simulink model "real_model_ctrl_2023a"  (R2024b)
settings: Solver=VariableStepAuto  StartTime=0.0  StopTime=1000  RelTol=1e-3
undefined symbols (not defined in the file or in its folder): National_Instruments, PCI
libraries: sldrtlib x3, slpidlib x1
settings Model: Creator=andit  LastModifiedBy=andit

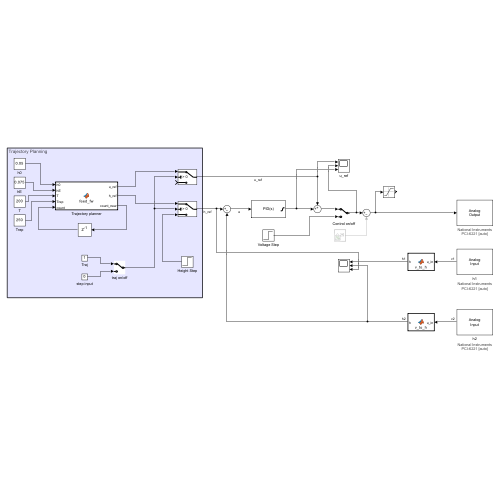
[thumbnail: Simulink's stored preview of the top-level diagram]
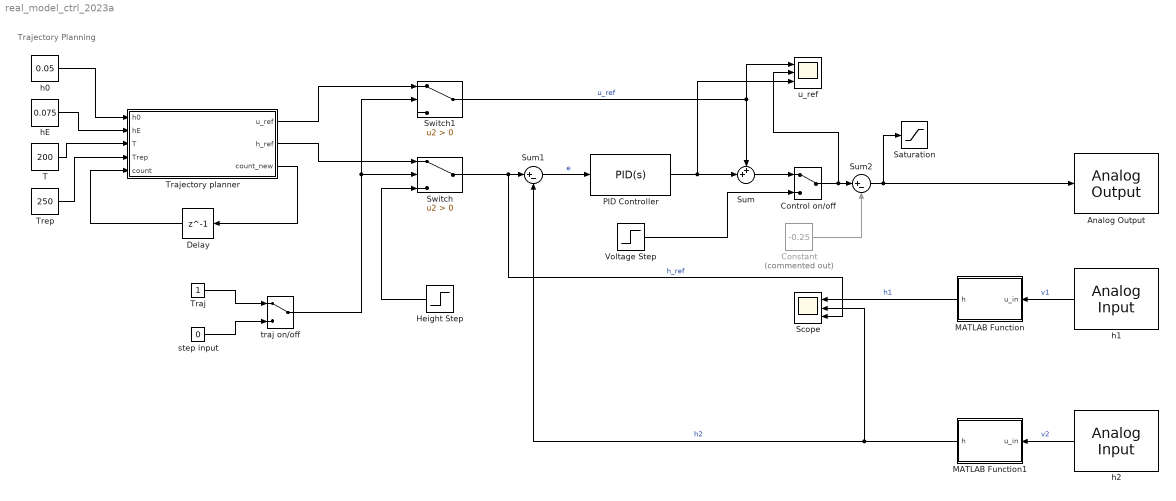
== system real_model_ctrl_2023a ==
  note: Trajectory Planning
  Analog Output : sldrtlib/Analog Output  SampleTime=0.1  MaxMissedTicks=10  ShowMissedTicks=off  YieldWhenWaiting=off  DrvName=National_Instruments/PCI-6221  DrvAddress=4294967295  DrvOptions=[0 1 0 0 0]  Channels=1  RangeMode=1  VoltRange=1  InitialValue=[]  FinalValue=[]
      settings: AttributesFormatString=National Instruments\nPCI-6221 [auto]
  Constant : Constant  Commented=on  Value=-0.25
  Control on/off : ManualSwitch
  Delay : Delay  DelayLength=1
  Height Step : Step  After=50  SampleTime=0
  MATLAB Function : MATLAB Function  TreatAsAtomicUnit=on
  MATLAB Function1 : MATLAB Function  TreatAsAtomicUnit=on
  PID Controller : slpidlib/PID Controller  Controller=PID  Form=Parallel  TimeDomain=Continuous-time  UseExternalTs=off  SampleTime=-1  IntegratorMethod=Forward Euler  FilterMethod=Forward Euler  ControllerParametersSource=internal  P=20  I=5  UseKiTs=off  D=-0.145290491513972  UseExternalDerivativeSource=off  N=13.0234851937353  UseFilter=on  TunerSelectOption=Transfer Function Based (PID Tuner App)  InitialConditionSource=internal  InitialConditionForIntegrator=0  InitialConditionForFilter=0  DifferentiatorICPrevScaledInput=0  ExternalReset=none  TrackingMode=off  Kt=1  LimitOutput=on  SatLimitsSource=internal  UpperSaturationLimit=5  LowerSaturationLimit=0  LinearizeAsGain=on  AntiWindupMode=clamping  Kb=1  LimitIntegrator=off  UpperIntegratorSaturationLimit=inf  LowerIntegratorSaturationLimit=-inf  POutMin=[]  POutMax=[]  IOutMin=[]  IOutMax=[]  DOutMin=[]  DOutMax=[]  NOutMin=[]  NOutMax=[]  SumOutMin=[]  SumOutMax=[]  SaturationOutMin=[]  SaturationOutMax=[]  PParamMin=[]  PParamMax=[]  IParamMin=[]  IParamMax=[]  DParamMin=[]  DParamMax=[]  NParamMin=[]  NParamMax=[]  KbParamMin=[]  KbParamMax=[]  KtParamMin=[]  KtParamMax=[]  KbOutMin=[]  KbOutMax=[]  KtOutMin=[]  KtOutMax=[]  IntegratorOutMin=[]  IntegratorOutMax=[]  FilterOutMin=[]  FilterOutMax=[]  SumI1OutMin=[]  SumI1OutMax=[]  SumI2OutMin=[]  SumI2OutMax=[]  SumI3OutMin=[]  SumI3OutMax=[]  SumI4OutMin=[]  SumI4OutMax=[]  SumDOutMin=[]  SumDOutMax=[]  DifferentiatorOutMin=[]  DifferentiatorOutMax=[]  FilterDiffOutCoefMin=[]  FilterDiffOutCoefMax=[]  ReciprocalOutMin=[]  ReciprocalOutMax=[]  SumDenOutMin=[]  SumDenOutMax=[]  SumNumOutMin=[]  SumNumOutMax=[]  DivideOutMin=[]  DivideOutMax=[]  UdiffTsProdOutMin=[]  UdiffTsProdOutMax=[]  NTsProdOutMin=[]  NTsProdOutMax=[]  UintegralTsProdOutMin=[]  UintegralTsProdOutMax=[]  UngainTsProdOutMin=[]  UngainTsProdOutMax=[]  ClampingZeroOutDataTypeStr=Inherit: Inherit via back propagation  ClampingZeroOutMin=[]  ClampingZeroOutMax=[]  FilterDenConstantOutDataTypeStr=Inherit: Inherit via back propagation  FilterDenConstantOutMin=[]  FilterDenConstantOutMax=[]  PCopyOutDataTypeStr=Inherit: Inherit via back propagation  PCopyOutMin=[]  PCopyOutMax=[]  NCopyOutDataTypeStr=Inherit: Inherit via back propagation  NCopyOutMin=[]  NCopyOutMax=[]  IntegratorContinuousStateAttributes=''  IntegratorStateMustResolveToSignalObject=off  IntegratorRTWStateStorageClass=Auto  FilterContinuousStateAttributes=''  FilterStateMustResolveToSignalObject=off  FilterRTWStateStorageClass=Auto  ParallelPVariant=InternalParameters  IdealPVariant=Disabled  IVariant=InternalParameters  DVariant=InternalParameters  IntegratorVariant=Continuous  SatVariant=Enabled  AWVariant=ContClampingParallel  PCopyVariant=Disabled  TRVariant=Disabled  FdbkBlocksVariant=Forward  IdealPFdbkVariant=Disabled  SatFdbkVariant=Disabled  DerivativeFilterVariant=ContFilter  NVariant=InternalParameters  NCopyVariant=Disabled  FilterICVariant=InternalICsFilter  IntegratorICVariant=InternalICs  ExternalResetVariant=Disabled  TRSumVariant=Passthrough  SumFdbkVariant=Disabled  SumVariant=Sum_PID  TsampFilterVariant=InternalTs  TsampNgainVariant=Passthrough  TsampIntegralVariant=Disabled_SignalSpec  ExternalSaturationOutDataTypeStr=Inherit: Same as second input  DerivativeSourceVariant=ErrorSignal  PreIntVariant=InternalPreInt
  Saturation : Saturate  UpperLimit=5  LowerLimit=0
  Scope : Scope  NumInputPorts=3
  Sum : Sum  Inputs=++|
  Sum1 : Sum  Inputs=|+-
  Sum2 : Sum  Inputs=|+-
  Switch : Switch  Criteria=u2 > Threshold  SaturateOnIntegerOverflow=off  InputSameDT=off
  Switch1 : Switch  Criteria=u2 > Threshold  SaturateOnIntegerOverflow=off  InputSameDT=off
  T : Constant  Value=200
  Traj : Constant
  Trajectory planner : MATLAB Function  TreatAsAtomicUnit=on
  Trep : Constant  Value=250
  Voltage Step : Step  Time=0  After=0  SampleTime=0
  h0 : Constant  Value=0.05
  h1 : sldrtlib/Analog Input  SampleTime=0.1  MaxMissedTicks=10  ShowMissedTicks=off  YieldWhenWaiting=off  DrvName=National_Instruments/PCI-6221  DrvAddress=4294967295  DrvOptions=[0 1 0 0 0]  Channels=1  RangeMode=1  VoltRange=1  DataType=1
      settings: AttributesFormatString=National Instruments\nPCI-6221 [auto]
  h2 : sldrtlib/Analog Input  SampleTime=0.1  MaxMissedTicks=10  ShowMissedTicks=off  YieldWhenWaiting=off  DrvName=National_Instruments/PCI-6221  DrvAddress=4294967295  DrvOptions=[0 1 0 0 0]  Channels=2  RangeMode=1  VoltRange=1  DataType=1
      settings: AttributesFormatString=National Instruments\nPCI-6221 [auto]
  hE : Constant  Value=0.075
  step input : Constant  Value=0
  traj on/off : ManualSwitch
  u_ref : Scope  NumInputPorts=3
  wires:
  h1/1 -> MATLAB Function/1(u_in)  "v1"
  Sum1/1 -> PID Controller/1  "e"
  PID Controller/1 -> u_ref/3, Sum/2
  h0/1 -> Trajectory planner/1(h0)
  Delay/1 -> Trajectory planner/5(count)
  traj on/off/1 -> Switch/2, Switch1/2
  hE/1 -> Trajectory planner/2(hE)
  step input/1 -> traj on/off/2
  Sum/1 -> Control on/off/1
  Voltage Step/1 -> Control on/off/2
  Trajectory planner/2(h_ref) -> Switch/1
  Traj/1 -> traj on/off/1
  Switch1/1 -> u_ref/1, Sum/1  "u_ref"
  Switch/1 -> Scope/3, Sum1/1  "h_ref"
  Trajectory planner/1(u_ref) -> Switch1/1
  Trajectory planner/3(count_new) -> Delay/1
  Height Step/1 -> Switch/3
  h2/1 -> MATLAB Function1/1(u_in)  "v2"
  MATLAB Function1/1(h) -> Sum1/2, Scope/2  "h2"
  MATLAB Function/1(h) -> Scope/1  "h1"
  Sum2/1 -> Analog Output/1, Saturation/1
  Control on/off/1 -> u_ref/2, Sum2/1
  Constant/1 -> Sum2/2
  Trep/1 -> Trajectory planner/4(Trep)
  T/1 -> Trajectory planner/3(T)

== matlab function real_model_ctrl_2023a/Trajectory planner ==
  data: u_ref output; h_ref output; h0 input; hE input; T input; Trep input; count input; count_new output
function [u_ref, h_ref, count_new] = feed_fw(h0, hE, T, Trep, count)

count_new = count+1;
dT = 0.1;
t = count_new*dT;

if mod(floor(t/Trep), 2)
    h0_traj = h0;
    hE_traj = hE;
else
    h0_traj = hE;
    hE_traj = h0;
end

rho = 997;
A_t = 5e-5; % m^2
K_pump = 0.016666666700000;
u0 = 1/4; % V

a = 1.540430976133678;


x_dot = 0;

tau = rem(t, Trep);

if tau > T
    x_ref = hE_traj;
else
    Dh = hE_traj - h0_traj;
    a0 = h0_traj;
    a1 = 0;
    a2 = 3*Dh / T^2;
    a3 = -2*Dh / T^3;

    x_ref = a0 + a1*tau + a2*tau^2 + a3*tau^3;
    x_dot = a1 + 2*a2*tau + 3*a3*tau^2;
    
end

h_ref = x_ref;
u_ref = (x_dot + a*sqrt(x_ref))*rho*A_t / (K_pump) + u0; % Sprung im U-ref?
end

== matlab function real_model_ctrl_2023a/MATLAB Function ==
  data: u_in input; h output
function h  = v_to_h(u_in)
    h = 0.1254.*u_in - 0.2682;
end

== matlab function real_model_ctrl_2023a/MATLAB Function1 ==
  data: u_in input; h output
function h  = v_to_h(u_in)
    h = 0.1254.*u_in - 0.2682;
end
